simulink model "Three_Phase_Full_Wave_Full_Conrolled_Bridge_Rectifier_RL_Load"  (R2018a)
settings: Solver=VariableStepAuto  StartTime=0.0  StopTime=0.1  RelTol=1e-3
libraries: powerlib x31, powerlib_meascontrol x5
settings Model: Creator=ozie  LastModifiedBy=ozie

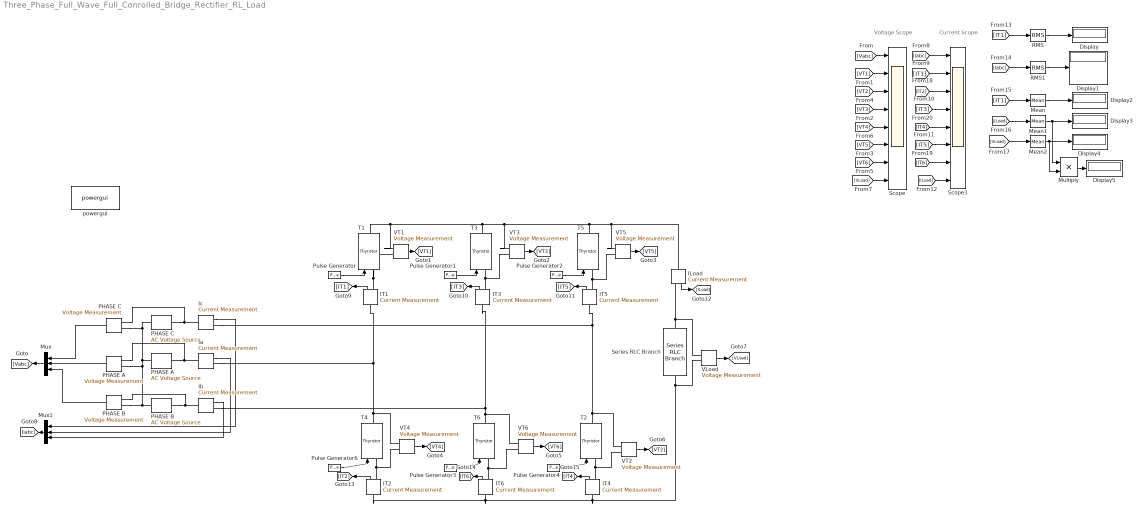
== system Three_Phase_Full_Wave_Full_Conrolled_Bridge_Rectifier_RL_Load ==
  note: Current Scope
  note: Voltage Scope
  Display{,1..5} (6 alike) : Display
  ILoad : powerlib/Measurements/Current Measurement  PhasorSimulation=off  OutputType=Complex  PSBequivalent=0
  IT{1..5} (5 alike) : powerlib/Measurements/Current Measurement  PhasorSimulation=off  OutputType=Complex  PSBequivalent=0
  "IT6 " : powerlib/Measurements/Current Measurement  PhasorSimulation=off  OutputType=Complex  PSBequivalent=0
  Ia : powerlib/Measurements/Current Measurement  PhasorSimulation=off  OutputType=Complex  PSBequivalent=0
  Ib : powerlib/Measurements/Current Measurement  PhasorSimulation=off  OutputType=Complex  PSBequivalent=0
  Ic : powerlib/Measurements/Current Measurement  PhasorSimulation=off  OutputType=Complex  PSBequivalent=0
  Mean : powerlib_meascontrol/Measurements/Mean  Freq=60  Vinit=0  Ts=0
  Mean1 : powerlib_meascontrol/Measurements/Mean  Freq=60  Vinit=0  Ts=0
  Mean2 : powerlib_meascontrol/Measurements/Mean  Freq=60  Vinit=0  Ts=0
  Multiply : Product
  Mux : Mux  Inputs=3
      settings: DisplayOption=signals
  Mux1 : Mux  Inputs=3
      settings: DisplayOption=signals
  PHASE A : powerlib/Electrical Sources/AC Voltage Source  Amplitude=220*sqrt(2)  Phase=0  Frequency=50  SampleTime=0  Measurements=None  BusType=swing  Pref=10e3  Qref=0  Qmin=-inf  Qmax=+inf
  "PHASE A " : powerlib/Measurements/Voltage Measurement  PhasorSimulation=off  OutputType=Complex  PSBequivalent=0
  PHASE B : powerlib/Electrical Sources/AC Voltage Source  Amplitude=220*sqrt(2)  Phase=120  Frequency=50  SampleTime=0  Measurements=None  BusType=swing  Pref=10e3  Qref=0  Qmin=-inf  Qmax=+inf
  "PHASE B " : powerlib/Measurements/Voltage Measurement  PhasorSimulation=off  OutputType=Complex  PSBequivalent=0
  PHASE C : powerlib/Electrical Sources/AC Voltage Source  Amplitude=220*sqrt(2)  Phase=-120  Frequency=50  SampleTime=0  Measurements=None  BusType=swing  Pref=10e3  Qref=0  Qmin=-inf  Qmax=+inf
  "PHASE C " : powerlib/Measurements/Voltage Measurement  PhasorSimulation=off  OutputType=Complex  PSBequivalent=0
  Pulse Generator : DiscretePulseGenerator  PulseType=Time based  Period=1/50  PulseWidth=5  PhaseDelay=0.01*(120/360)
  Pulse Generator1 : DiscretePulseGenerator  PulseType=Time based  Period=1/50  PulseWidth=5  PhaseDelay=0.01*(240/360)
  Pulse Generator2 : DiscretePulseGenerator  PulseType=Time based  Period=1/50  PulseWidth=5  PhaseDelay=0.01*(360/360)
  Pulse Generator3 : DiscretePulseGenerator  PulseType=Time based  TimeSource=Use external signal  Period=1/50  PulseWidth=5  PhaseDelay=0.01*(60/360)
  Pulse Generator4 : DiscretePulseGenerator  PulseType=Time based  Period=1/50  PulseWidth=5  PhaseDelay=0.01*(180/360)
  Pulse Generator6 : DiscretePulseGenerator  PulseType=Time based  Period=1/50  PulseWidth=5  PhaseDelay=0.01*(300/360)
  RMS : powerlib_meascontrol/Measurements/RMS  TrueRMS=on  Freq=50  RMSInit=120  Ts=0
  RMS1 : powerlib_meascontrol/Measurements/RMS  TrueRMS=on  Freq=50  RMSInit=120  Ts=0
  Scope : Scope  NumInputPorts=8
  Scope1 : Scope  NumInputPorts=8
  Series RLC Branch : powerlib/Elements/Series RLC Branch  LConnTagsString=__new0  RConnTagsString=__new0  BranchType=RL  Resistance=10  Inductance=10e-3  SetiL0=off  InitialCurrent=0  Capacitance=1e-6  Setx0=off  InitialVoltage=0  Measurements=None
  T{1..6} (6 alike) : powerlib/Power Electronics/Thyristor  Ron=0.001  Lon=0  Vf=0.8  IC=0  Rs=1e6  Cs=250e-9  Measurements=off
  VLoad : powerlib/Measurements/Voltage Measurement  PhasorSimulation=off  OutputType=Complex  PSBequivalent=0
  "VT1 " : powerlib/Measurements/Voltage Measurement  PhasorSimulation=off  OutputType=Complex  PSBequivalent=0
  "VT2 " : powerlib/Measurements/Voltage Measurement  PhasorSimulation=off  OutputType=Complex  PSBequivalent=0
  "VT3 " : powerlib/Measurements/Voltage Measurement  PhasorSimulation=off  OutputType=Complex  PSBequivalent=0
  "VT4 " : powerlib/Measurements/Voltage Measurement  PhasorSimulation=off  OutputType=Complex  PSBequivalent=0
  "VT5 " : powerlib/Measurements/Voltage Measurement  PhasorSimulation=off  OutputType=Complex  PSBequivalent=0
  "VT6 " : powerlib/Measurements/Voltage Measurement  PhasorSimulation=off  OutputType=Complex  PSBequivalent=0
  powergui : powerlib/powergui  Priority=1  SimulationMode=Continuous  SampleTime=50e-6  frequency=60  Iterations=50  frequencyindice=50  Pbase=100e6  ErrMax=1e-4  UnitsV=kV  UnitsW=MW  buscounter=0  FunctionMessages=off  echomessages=off  EnableUseOfTLC=off  CurrentSourceSwitches=off  DisableSnubberDevices=off  DisableRonSwitches=off  DisableVfSwitches=off  DisplayEquations=off  SolverType=Tustin/Backward Euler (TBE)  Interpol=off  ExternalGateDelay=off  methode=off  Ts=100  x0status=blocks  SPID=on  SwTol=0  HookPort=off  RestoreLinks=warning  ResistiveCurrentMeasurement=off  Frange=[0:2:500]  Ylog=off  Xlog=on  ShowGrid=off  save=off  variable=ZData  structure=0  ZoomFFT=off  StartTime=0.0  cycles=1  DisplayStyle=1  fundamental=60  FreqAxis=off  MaxFrequency=1000  frequencyindicesteady=1  RmsSteady=1  display=off
  wires:
  "PHASE C "/1 -> Mux/1
  "PHASE A "/1 -> Mux/2
  "PHASE B "/1 -> Mux/3
  Pulse Generator/1 -> T1/1
  Pulse Generator1/1 -> T3/1
  Pulse Generator2/1 -> T5/1
  Pulse Generator4/1 -> T2/1
  Pulse Generator3/1 -> T6/1
  Pulse Generator6/1 -> T4/1
  Mux/1 -> [Vabc]
  "VT1 "/1 -> [VT1]
  "VT3 "/1 -> [VT3]
  "VT5 "/1 -> [VT5]
  "VT4 "/1 -> [VT4]
  "VT6 "/1 -> [VT6]
  "VT2 "/1 -> [VT2]
  [Vabc] -> Scope/1
  [VT1] -> Scope/2
  [VT2] -> Scope/3
  [VT3] -> Scope/4
  [VT4] -> Scope/5
  [VT5] -> Scope/6
  [VT6] -> Scope/7
  VLoad/1 -> [VLoad]
  [VLoad] -> Scope/8
  Ic/1 -> Mux1/1
  Ia/1 -> Mux1/2
  Ib/1 -> Mux1/3
  Mux1/1 -> [Iabc]
  IT1/1 -> [IT1]
  IT3/1 -> [IT3]
  IT5/1 -> [IT5]
  ILoad/1 -> [ILoad]
  [IT1] -> RMS/1
  RMS/1 -> Display/1
  [Iabc] -> RMS1/1
  RMS1/1 -> Display1/1
  [IT1] -> Mean/1
  Mean/1 -> Display2/1
  Mean1/1 -> Display3/1, Multiply/1
  [ILoad] -> Mean1/1
  Mean2/1 -> Display4/1, Multiply/2
  [VLoad] -> Mean2/1
  Multiply/1 -> Display5/1
  IT2/1 -> [IT2]
  "IT6 "/1 -> [IT6]
  IT4/1 -> [IT4]
  [Iabc] -> Scope1/1
  [IT1] -> Scope1/2
  [IT2] -> Scope1/3
  [IT3] -> Scope1/4
  [IT4] -> Scope1/5
  [IT5] -> Scope1/6
  [IT6] -> Scope1/7
  [ILoad] -> Scope1/8
  connections:
  PHASE C/LConn1 -- "PHASE C "/LConn2 -- PHASE A/LConn1 -- "PHASE B "/LConn2 -- PHASE B/LConn1 -- "PHASE A "/LConn2
  PHASE A/RConn1 -- "PHASE A "/LConn1 -- Ia/LConn1
  T3/LConn1 -- "VT3 "/LConn1 -- IT3/RConn1
  T5/LConn1 -- "VT5 "/LConn1 -- IT5/RConn1
  T1/RConn1 -- ILoad/LConn1 -- "VT5 "/LConn2 -- T5/RConn1 -- "VT3 "/LConn2 -- T3/RConn1 -- "VT1 "/LConn2
  T2/LConn1 -- IT4/RConn1 -- "VT2 "/LConn1
  "PHASE C "/LConn1 -- Ic/LConn1 -- PHASE C/RConn1
  T1/LConn1 -- IT1/RConn1 -- "VT1 "/LConn1
  "PHASE B "/LConn1 -- Ib/LConn1 -- PHASE B/RConn1
  Ia/RConn1 -- "VT4 "/LConn2 -- T4/RConn1 -- IT1/LConn1
  "VT6 "/LConn2 -- T6/RConn1 -- IT3/LConn1 -- Ib/RConn1
  Ic/RConn1 -- IT5/LConn1 -- "VT2 "/LConn2 -- T2/RConn1
  VLoad/LConn1 -- ILoad/RConn1 -- Series RLC Branch/RConn1
  "VT4 "/LConn1 -- T4/LConn1 -- IT2/RConn1
  "VT6 "/LConn1 -- "IT6 "/RConn1 -- T6/LConn1
  IT2/LConn1 -- "IT6 "/LConn1 -- VLoad/LConn2 -- Series RLC Branch/LConn1 -- IT4/LConn1
